simulink model "Model"  (R2024a)
settings: Solver=VariableStepAuto  StartTime=0.0  StopTime=20  MaxStep=0.1  RelTol=1e-3
values from neighbouring files (symbols this model uses):
  Ae = [-k/m 0 1/m; 1 0 0; 0 0 0]    [Analysis.m]
  Be = [1/m; 0; 0]    [Analysis.m]
  C_L_d = c2d(C_L, Ts, 'matched')    [Analysis.m]
  Ce = [0 1 0]    [Analysis.m]
  k = 0.5    [Analysis.m]
  L = place(Ae', Ce', [-3 -3.5 -4])'    [Analysis.m]
  m = 10    [Analysis.m]
  Ts = 0.1    [Analysis.m]
undefined symbols (not defined in the file or in its folder): DiscIntNeverNeededParam
libraries: simulink x1
settings Model: Creator=berto  LastModifiedBy=berto

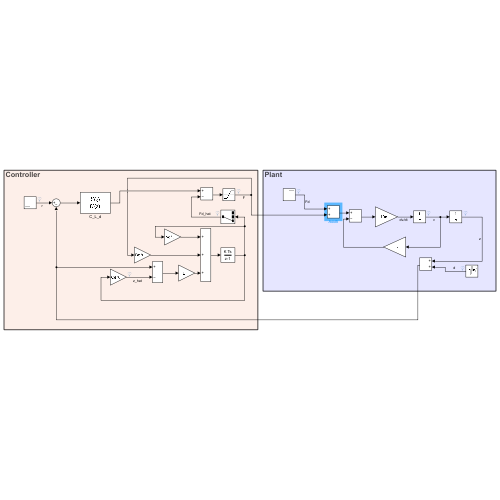
[thumbnail: Simulink's stored preview of the top-level diagram]
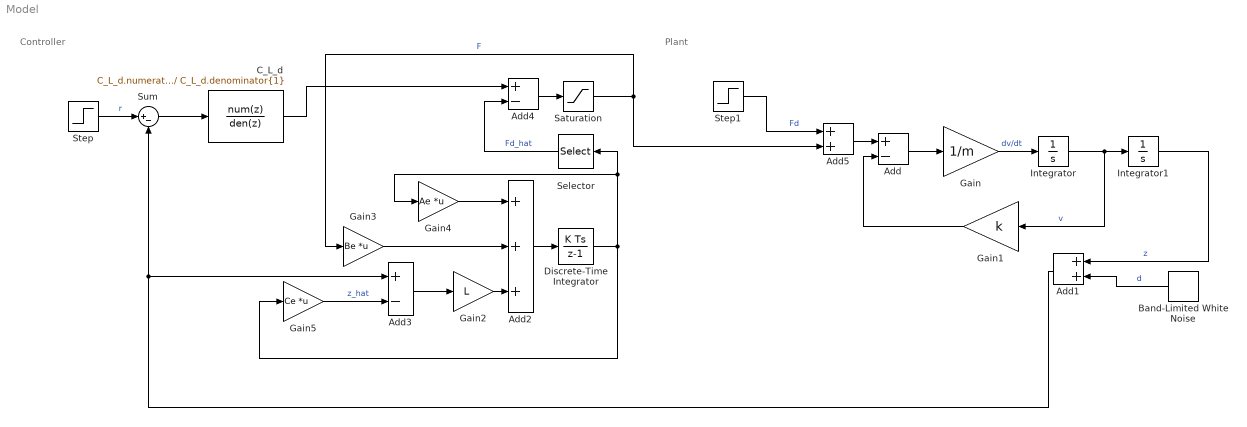
== system Model ==
  note: Controller
  note: Plant
  Add : Sum  Inputs=+-
  Add1 : Sum
  Add2 : Sum  Inputs=+++
  Add3 : Sum  Inputs=+-
  Add4 : Sum  Inputs=+-
  Add5 : Sum
  Band-Limited White Noise : simulink/Sources/Band-Limited White Noise  Cov=[0.00001]  Ts=0.1  seed=[23341]
  C_L_d : DiscreteTransferFcn  Numerator=C_L_d.numerator{1}  Denominator=C_L_d.denominator{1}
  Discrete-Time Integrator : DiscreteIntegrator  SampleTime=Ts  ICPrevOutput=DiscIntNeverNeededParam  ICPrevScaledInput=DiscIntNeverNeededParam
  Gain : Gain  Gain=1/m
  Gain1 : Gain  Gain=k
  Gain2 : Gain  Gain=L
  Gain3 : Gain  Gain=Be  Multiplication=Matrix(K*u)
  Gain4 : Gain  Gain=Ae  Multiplication=Matrix(K*u)
  Gain5 : Gain  Gain=Ce  Multiplication=Matrix(K*u)
  Integrator : Integrator
  Integrator1 : Integrator
  Saturation : Saturate  UpperLimit=50  LowerLimit=-50
  Selector : Selector  InputPortWidth=3  IndexOptions=Index vector (dialog)  Indices=[3]  OutputSizes=1
  Step : Step  SampleTime=Ts
  Step1 : Step  Time=10  After=20  SampleTime=0
  Sum : Sum  Inputs=|+-
  wires:
  C_L_d/1 -> Add4/1
  Step/1 -> Sum/1  "r"
  Sum/1 -> C_L_d/1
  Integrator1/1 -> Add1/1  "z"
  Add/1 -> Gain/1
  Gain/1 -> Integrator/1  "dv/dt"
  Integrator/1 -> Gain1/1, Integrator1/1  "v"
  Gain1/1 -> Add/2
  Band-Limited White Noise/1 -> Add1/2  "d"
  Add1/1 -> Add3/1, Sum/2
  Add2/1 -> Discrete-Time Integrator/1
  Gain3/1 -> Add2/2
  Gain4/1 -> Add2/1
  Discrete-Time Integrator/1 -> Gain5/1, Selector/1, Gain4/1
  Gain2/1 -> Add2/3
  Add3/1 -> Gain2/1
  Gain5/1 -> Add3/2  "z_hat"
  Selector/1 -> Add4/2  "Fd_hat"
  Add5/1 -> Add/1
  Add4/1 -> Saturation/1
  Saturation/1 -> Gain3/1, Add5/2  "F"
  Step1/1 -> Add5/1  "Fd"
